simulink model "Problem_3"  (R2020a)
settings: Solver=ode45  StartTime=0.0  StopTime=10  RelTol=1e-3
PreLoadFcn:
  | b=50;
  | m1 = 2500;
  | m2 = 320;
  | k1 = 50000;
  | k2 = 50000;
  | b1 = 350;
  | u=500;
  | m=1000;
undefined symbols (not defined in the file): sigbuilder_block
libraries: simulink x1
settings Model: Creator=Ganesh  LastModifiedBy=Ganesh

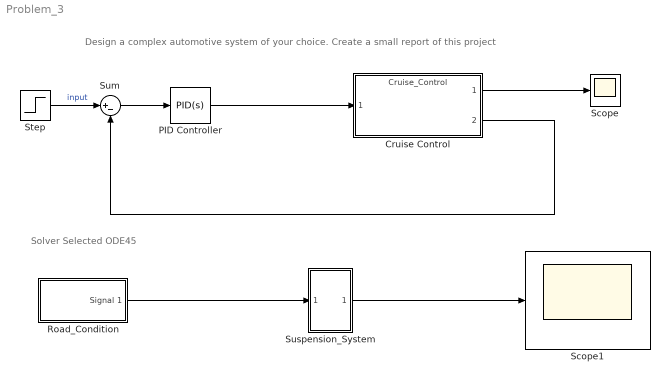
== system Problem_3 ==
  note: Solver Selected ODE45
  note: Design a complex automotive system of your choice. Create a small report of this project
  Cruise Control : ModelReference  ModelNameDialog=Cruise_Control  ModelReferenceVersion=1.8
  PID Controller : simulink/Continuous/PID Controller  Controller=PID  Form=Parallel  TimeDomain=Continuous-time  UseExternalTs=off  SampleTime=-1  IntegratorMethod=Forward Euler  FilterMethod=Forward Euler  ControllerParametersSource=internal  P=62.2621857990546  I=35.6695644082268  D=-3.39221410169137  UseFilter=on  N=4.29513847523714  TunerSelectOption=Transfer Function Based (PID Tuner App)  InitialConditionSource=internal  InitialConditionForIntegrator=0  InitialConditionForFilter=0  DifferentiatorICPrevScaledInput=0  ExternalReset=none  TrackingMode=off  Kt=1  LimitOutput=off  UpperSaturationLimit=inf  LowerSaturationLimit=-inf  LinearizeAsGain=on  AntiWindupMode=none  Kb=1  POutMin=[]  POutMax=[]  IOutMin=[]  IOutMax=[]  DOutMin=[]  DOutMax=[]  NOutMin=[]  NOutMax=[]  SumOutMin=[]  SumOutMax=[]  SaturationOutMin=[]  SaturationOutMax=[]  PParamMin=[]  PParamMax=[]  IParamMin=[]  IParamMax=[]  DParamMin=[]  DParamMax=[]  NParamMin=[]  NParamMax=[]  KbParamMin=[]  KbParamMax=[]  KtParamMin=[]  KtParamMax=[]  KbOutMin=[]  KbOutMax=[]  KtOutMin=[]  KtOutMax=[]  IntegratorOutMin=[]  IntegratorOutMax=[]  FilterOutMin=[]  FilterOutMax=[]  SumI1OutMin=[]  SumI1OutMax=[]  SumI2OutMin=[]  SumI2OutMax=[]  SumI3OutMin=[]  SumI3OutMax=[]  SumI4OutMin=[]  SumI4OutMax=[]  SumDOutMin=[]  SumDOutMax=[]  DifferentiatorOutMin=[]  DifferentiatorOutMax=[]  FilterDiffOutCoefMin=[]  FilterDiffOutCoefMax=[]  ReciprocalOutMin=[]  ReciprocalOutMax=[]  SumDenOutMin=[]  SumDenOutMax=[]  SumNumOutMin=[]  SumNumOutMax=[]  DivideOutMin=[]  DivideOutMax=[]  UdiffTsProdOutMin=[]  UdiffTsProdOutMax=[]  NTsProdOutMin=[]  NTsProdOutMax=[]  UintegralTsProdOutMin=[]  UintegralTsProdOutMax=[]  UngainTsProdOutMin=[]  UngainTsProdOutMax=[]  IntegratorContinuousStateAttributes=''  IntegratorStateMustResolveToSignalObject=off  IntegratorRTWStateStorageClass=Auto  FilterContinuousStateAttributes=''  FilterStateMustResolveToSignalObject=off  FilterRTWStateStorageClass=Auto  ParallelPVariant=InternalParameters  IdealPVariant=Disabled  IVariant=InternalParameters  DVariant=InternalParameters  IntegratorVariant=Continuous  SatVariant=Disabled  AWVariant=Passthrough  PCopyVariant=Disabled  TRVariant=Disabled  FdbkBlocksVariant=Forward  IdealPFdbkVariant=Disabled  SatFdbkVariant=Disabled  DerivativeFilterVariant=ContFilter  NVariant=InternalParameters  NCopyVariant=Disabled  FilterICVariant=InternalICsFilter  IntegratorICVariant=InternalICs  ExternalResetVariant=Disabled  TRSumVariant=Passthrough  SumFdbkVariant=Disabled  SumVariant=Sum_PID  TsampFilterVariant=InternalTs  TsampNgainVariant=Passthrough  TsampIntegralVariant=Passthrough
  Road_Condition : Subsystem  Tag=STV Subsys  LoadFcn=sigbuilder_block('load');  StartFcn=sigbuilder_block('start');  StopFcn=sigbuilder_block('stop');  ClipboardFcn=sigbuilder_block('clipboard');  mask(Sigbuilder block){tuvar=[0:10]}
      mask help: Simulink:masks:SigbuilderBlock_MD
      mask init:
      | if ~strcmp(get_param(bdroot(gcbh),'SimulationStatus'),'stopped') tuvar = sigbuilder_block('maskInit'); end
      settings: CopyFcn=sigbuilder_block('copy');  DeleteFcn=sigbuilder_block('delete');  ModelCloseFcn=sigbuilder_block('modelClose');  PreSaveFcn=sigbuilder_block('preSave');  PauseFcn=sigbuilder_block('pause');  ContinueFcn=sigbuilder_block('continue');  NameChangeFcn=sigbuilder_block('namechange');  OpenFcn=sigbuilder_block('open',[437.6 199.2 550.4 400 ]);  CloseFcn=sigbuilder_block('close');
      mask Display: plot(0, 0, 100, 100,[2, 2, 32, 32, 2], [68, 8, 8, 68, 68],[32, 2], [38, 38], [32, 19, 2],[53, 60, 44], [32, 17, 17, 2],[16, 16, 31, 31]);txt = getActiveGroup(gcbh);text(2, 100, txt,'verticalAlignment', 'top');
  Scope : Scope
  Scope1 : Scope
  Step : Step  Time=0  After=u  SampleTime=0
  Sum : Sum  Inputs=|+-
  Suspension_System : Subsystem
  wires:
  Cruise Control/1 -> Scope/1
  Sum/1 -> PID Controller/1
  PID Controller/1 -> Cruise Control/1
  Step/1 -> Sum/1  "input"
  Cruise Control/2 -> Sum/2
  Road_Condition/1(Signal 1) -> Suspension_System/1(In1)
  Suspension_System/1(Out1) -> Scope1/1

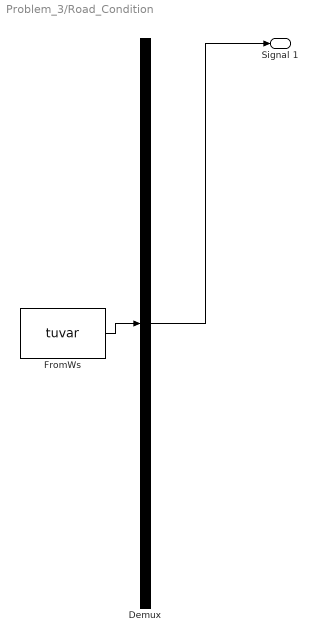
== system Problem_3/Road_Condition ==
  Demux : Demux  Tag=STV Demux  Outputs=1
      settings: DisplayOption=none
  FromWs : FromWorkspace  Tag=STV FromWs  VariableName=tuvar
      SigBuilderData=|
      | common.afterFinalStr = 'Extrapolate'
      | common.sampleTime = 0
      | dataSet.timeRange = [0 10]
      | dataSet.name = 'Group 1'
      | sbobj.Groups.Name = 'Group 1'
      | sbobj.Groups.Signals.Name = 'Signal 1'
      | sbobj.Groups.Signals.XData = [0 0.5 0.5 1.88 1.88 10]
      | sbobj.Groups.Signals.YData = [0.015 0.15 0.41 0.365 0.53 0.065]
  Signal 1 : Outport  Tag=STV Outport
  wires:
  Demux/1 -> Signal 1/1
  FromWs/1 -> Demux/1

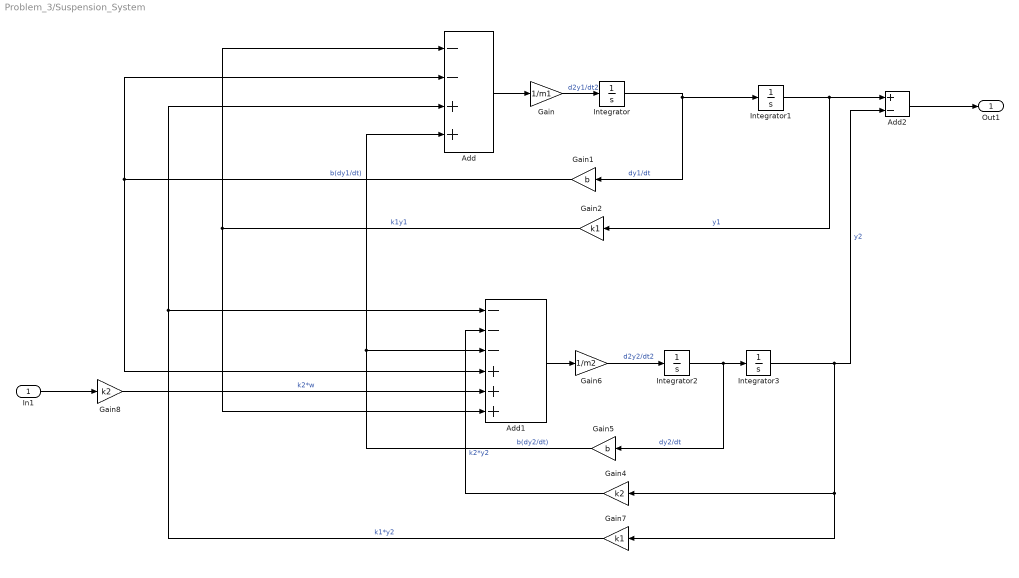
== system Problem_3/Suspension_System ==
  In1 : Inport
  Add : Sum  Inputs=--++
  Add1 : Sum  Inputs=---+++
  Add2 : Sum  Inputs=+-
  Gain : Gain  Gain=1/m1
  Gain1 : Gain  Gain=b
  Gain2 : Gain  Gain=k1
  Gain4 : Gain  Gain=k2
  Gain5 : Gain  Gain=b
  Gain6 : Gain  Gain=1/m2
  Gain7 : Gain  Gain=k1
  Gain8 : Gain  Gain=k2
  Integrator{,1..3} (4 alike) : Integrator
  Out1 : Outport
  wires:
  Add1/1 -> Gain6/1
  Gain7/1 -> Add/3, Add1/1  "k1*y2"
  Gain8/1 -> Add1/5  "k2*w"
  Add/1 -> Gain/1
  Gain1/1 -> Add/2, Add1/4  "b(dy1/dt)"
  Integrator2/1 -> Gain5/1, Integrator3/1  "dy2/dt"
  Integrator1/1 -> Add2/1, Gain2/1  "y1"
  Gain2/1 -> Add/1, Add1/6  "k1y1"
  Gain6/1 -> Integrator2/1  "d2y2/dt2"
  Integrator3/1 -> Gain7/1, Gain4/1, Add2/2  "y2"
  Gain/1 -> Integrator/1  "d2y1/dt2"
  In1/1 -> Gain8/1
  Gain5/1 -> Add/4, Add1/3  "b(dy2/dt)"
  Integrator/1 -> Integrator1/1, Gain1/1  "dy1/dt"
  Gain4/1 -> Add1/2  "k2*y2"
  Add2/1 -> Out1/1
